simulink model "windyBBBB_sim"  (R2022a)
settings: Solver=FixedStepDiscrete  StartTime=0.0  StopTime=40  FixedStep=0.01  RelTol=1e-3  EnableMultiTasking=on
undefined symbols (not defined in the file or in its folder): sigbuilder_block
libraries: simulink x12, simulink_extras x8
settings Model: PacingRate=0.100000  Creator=Lab  LastModifiedBy=Lab
settings SolverCC: AlgebraicLoopSolver=TrustRegion  AutoInsertRateTranBlk=on
settings DataIOCC: LimitDataPoints=on
settings OptimizationCC: LifeSpan=inf
settings DebuggingCC: UnconnectedInputMsg=warning  UnconnectedOutputMsg=warning  UnconnectedLineMsg=warning  AllowSymbolicDim=off  SFUnexpectedBacktrackingDiag=warning  SFNoUnconditionalDefaultTransitionDiag=warning  SFExecutionAtInitializationDiag=none  ArithmeticOperatorsInVariantConditions=warning
settings SFSimCC: SimUseLocalCustomCode=off  CustomCodeUndefinedFunction=UseInterfaceOnly
settings RTWCC: RTWUseLocalCustomCode=off  DLArmComputeVersion=19.05
settings CodeAppCC: StateflowObjectComments=on
settings GRTTargetCC: TargetLangStandard=C89/C90 (ANSI)
settings ConfigComp: CovMetricSettings=dw  CovSaveCumulativeToWorkspaceVar=on  CovSaveSingleToWorkspaceVar=on  CovExternalEMLEnable=off  CovSFcnEnable=off

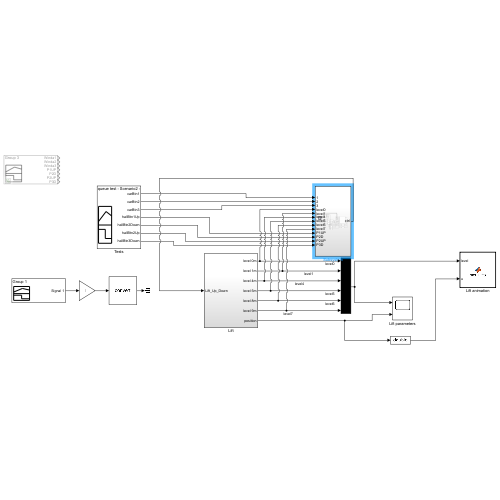
[thumbnail: Simulink's stored preview of the top-level diagram]
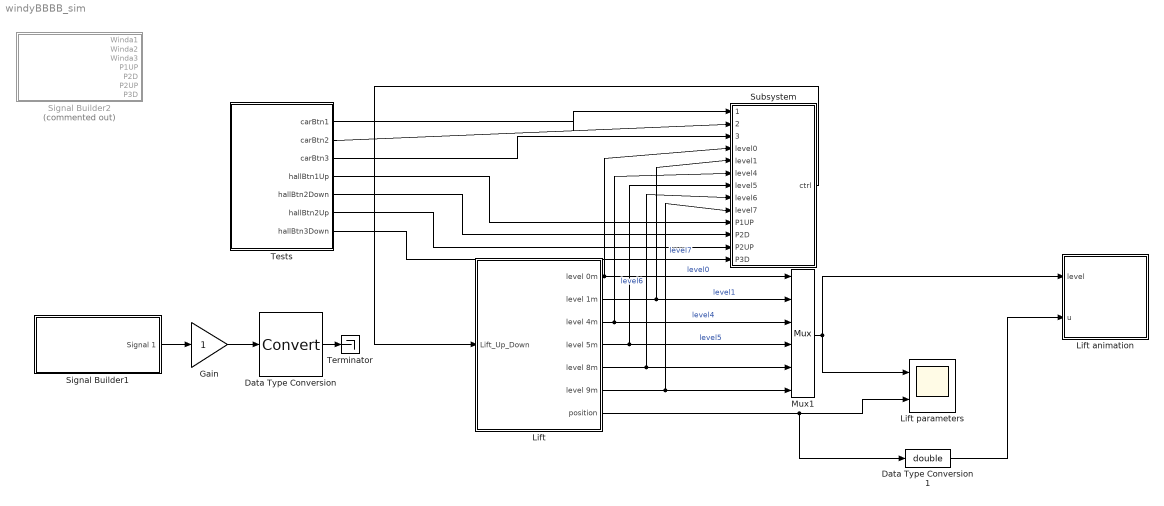
== system windyBBBB_sim ==
  Data Type Conversion : DataTypeConversion  SaturateOnIntegerOverflow=off  RndMeth=Floor
  Data Type Conversion1 : DataTypeConversion  OutDataTypeStr=double  SaturateOnIntegerOverflow=off  RndMeth=Floor
  Gain : Gain
  Lift : Subsystem
  Lift animation : MATLAB Function  TreatAsAtomicUnit=on  SystemSampleTime=0.05
  Lift parameters : Scope  NumInputPorts=2
  Mux1 : Mux  Inputs=6
  Signal Builder1 : Subsystem  Tag=STV Subsys  LoadFcn=sigbuilder_block('load');  StartFcn=sigbuilder_block('start');  StopFcn=sigbuilder_block('stop');  ClipboardFcn=sigbuilder_block('clipboard');  mask(Sigbuilder block){tuvar=[0:10]}
      mask help: Simulink:masks:SigbuilderBlock_MD
      mask init:
      | if ~strcmp(get_param(bdroot(gcbh),'SimulationStatus'),'stopped') tuvar = sigbuilder_block('maskInit'); end
      settings: CopyFcn=sigbuilder_block('copy');  DeleteFcn=sigbuilder_block('delete');  ModelCloseFcn=sigbuilder_block('modelClose');  PreSaveFcn=sigbuilder_block('preSave');  PauseFcn=sigbuilder_block('pause');  ContinueFcn=sigbuilder_block('continue');  NameChangeFcn=sigbuilder_block('namechange');  OpenFcn=sigbuilder_block('open',[327.75 241.5 550.5 394.5 ]);  CloseFcn=sigbuilder_block('close');
      mask Display: plot(0, 0, 100, 100,[2, 2, 32, 32, 2], [68, 8, 8, 68, 68],[32, 2], [38, 38], [32, 19, 2],[53, 60, 44], [32, 17, 17, 2],[16, 16, 31, 31]);txt = getActiveGroup(gcbh);text(2, 100, txt,'verticalAlignment', 'top');
  Signal Builder2 : Subsystem  Tag=STV Subsys  Commented=on  LoadFcn=sigbuilder_block('load');  StartFcn=sigbuilder_block('start');  StopFcn=sigbuilder_block('stop');  ClipboardFcn=sigbuilder_block('clipboard');  mask(Sigbuilder block){tuvar=[0:10]}
      mask help: Simulink:masks:SigbuilderBlock_MD
      mask init:
      | if ~strcmp(get_param(bdroot(gcbh),'SimulationStatus'),'stopped') tuvar = sigbuilder_block('maskInit'); end
      settings: CopyFcn=sigbuilder_block('copy');  DeleteFcn=sigbuilder_block('delete');  ModelCloseFcn=sigbuilder_block('modelClose');  PreSaveFcn=sigbuilder_block('preSave');  PauseFcn=sigbuilder_block('pause');  ContinueFcn=sigbuilder_block('continue');  NameChangeFcn=sigbuilder_block('namechange');  OpenFcn=sigbuilder_block('open',[-1440 -60 1440 723.6 ]);  CloseFcn=sigbuilder_block('close');
      mask Display: plot(0, 0, 100, 100,[2, 2, 32, 32, 2], [68, 8, 8, 68, 68],[32, 2], [38, 38], [32, 19, 2],[53, 60, 44], [32, 17, 17, 2],[16, 16, 31, 31]);txt = getActiveGroup(gcbh);text(2, 100, txt,'verticalAlignment', 'top');
  Subsystem : Subsystem
  Terminator : Terminator
  Tests : Subsystem  Tag=STV Subsys  LoadFcn=sigbuilder_block('load',[-1440 -60 1440 723.6 ]);  StartFcn=sigbuilder_block('start');  StopFcn=sigbuilder_block('stop');  ClipboardFcn=sigbuilder_block('clipboard');  mask(Sigbuilder block){tuvar=[0:10]}
      mask help: Simulink:masks:SigbuilderBlock_MD
      mask init:
      | if ~strcmp(get_param(bdroot(gcbh),'SimulationStatus'),'stopped') tuvar = sigbuilder_block('maskInit'); end
      settings: CopyFcn=sigbuilder_block('copy');  DeleteFcn=sigbuilder_block('delete');  ModelCloseFcn=sigbuilder_block('modelClose');  PreSaveFcn=sigbuilder_block('preSave');  PauseFcn=sigbuilder_block('pause');  ContinueFcn=sigbuilder_block('continue');  NameChangeFcn=sigbuilder_block('namechange');  OpenFcn=sigbuilder_block('open',[9.6 82.8 575.4 499.8 ]);  CloseFcn=sigbuilder_block('close');
      mask Display: plot(0, 0, 100, 100,[2, 2, 32, 32, 2], [68, 8, 8, 68, 68],[32, 2], [38, 38], [32, 19, 2],[53, 60, 44], [32, 17, 17, 2],[16, 16, 31, 31]);txt = getActiveGroup(gcbh);text(2, 100, txt,'verticalAlignment', 'top');
  wires:
  Lift/6(level 9m) -> Subsystem/9(level7), Mux1/6  "level7"
  Lift/2(level 1m) -> Subsystem/5(level1), Mux1/2  "level1"
  Data Type Conversion1/1 -> Lift animation/2(u)
  Lift/7(position) -> Data Type Conversion1/1, Lift parameters/2
  Mux1/1 -> Lift parameters/1, Lift animation/1(level)
  Lift/4(level 5m) -> Subsystem/7(level5), Mux1/4  "level5"
  Gain/1 -> Data Type Conversion/1
  Lift/5(level 8m) -> Subsystem/8(level6), Mux1/5  "level6"
  Signal Builder1/1(Signal 1) -> Gain/1
  Lift/1(level 0m) -> Subsystem/4(level0), Mux1/1  "level0"
  Lift/3(level 4m) -> Subsystem/6(level4), Mux1/3  "level4"
  Data Type Conversion/1 -> Terminator/1
  Tests/1(carBtn1) -> Subsystem/1(1)
  Tests/2(carBtn2) -> Subsystem/2(2)
  Tests/3(carBtn3) -> Subsystem/3(3)
  Subsystem/1(ctrl) -> Lift/1(Lift_Up_Down)
  Tests/4(hallBtn1Up) -> Subsystem/10(P1UP)
  Tests/5(hallBtn2Down) -> Subsystem/11(P2D)
  Tests/6(hallBtn2Up) -> Subsystem/12(P2UP)
  Tests/7(hallBtn3Down) -> Subsystem/13(P3D)

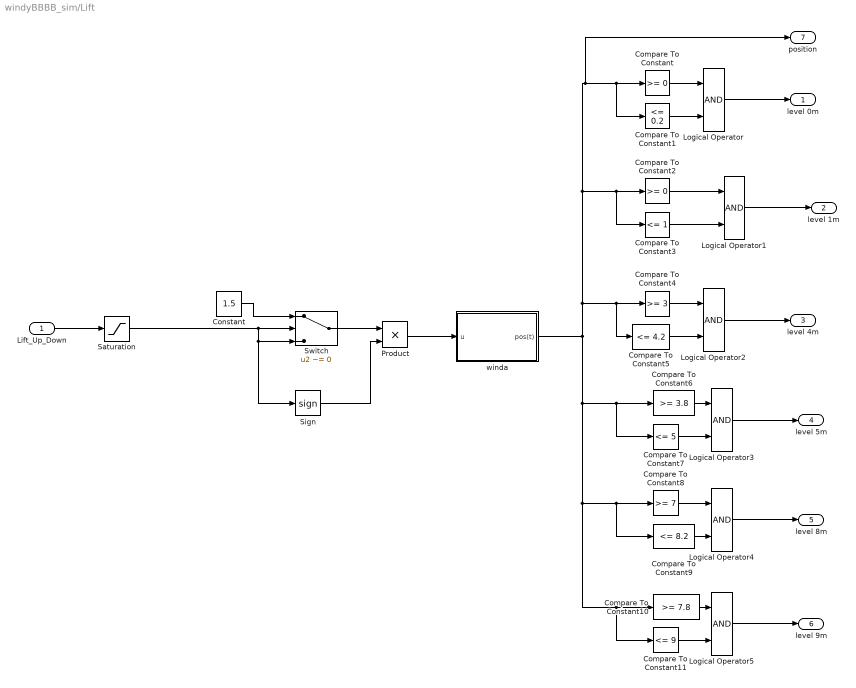
== system windyBBBB_sim/Lift ==
  Lift_Up_Down : Inport
  Compare To Constant : simulink/Logic and Bit Operations/Compare To Constant  relop=>=  const=0  OutDataTypeStr=boolean
  Compare To Constant1 : simulink/Logic and Bit Operations/Compare To Constant  relop=<=  const=0.2  OutDataTypeStr=boolean
  Compare To Constant10 : simulink/Logic and Bit Operations/Compare To Constant  relop=>=  const=7.8  OutDataTypeStr=boolean
  Compare To Constant11 : simulink/Logic and Bit Operations/Compare To Constant  relop=<=  const=9  OutDataTypeStr=boolean
  Compare To Constant2 : simulink/Logic and Bit Operations/Compare To Constant  relop=>=  const=0  OutDataTypeStr=boolean
  Compare To Constant3 : simulink/Logic and Bit Operations/Compare To Constant  relop=<=  const=1  OutDataTypeStr=boolean
  Compare To Constant4 : simulink/Logic and Bit Operations/Compare To Constant  relop=>=  const=3  OutDataTypeStr=boolean
  Compare To Constant5 : simulink/Logic and Bit Operations/Compare To Constant  relop=<=  const=4.2  OutDataTypeStr=boolean
  Compare To Constant6 : simulink/Logic and Bit Operations/Compare To Constant  relop=>=  const=3.8  OutDataTypeStr=boolean
  Compare To Constant7 : simulink/Logic and Bit Operations/Compare To Constant  relop=<=  const=5  OutDataTypeStr=boolean
  Compare To Constant8 : simulink/Logic and Bit Operations/Compare To Constant  relop=>=  const=7  OutDataTypeStr=boolean
  Compare To Constant9 : simulink/Logic and Bit Operations/Compare To Constant  relop=<=  const=8.2  OutDataTypeStr=boolean
  Constant : Constant  Value=1.5
  Logical Operator{,1..5} (6 alike) : Logic  AllPortsSameDT=off  OutDataTypeStr=boolean
  Product : Product  OutDataTypeStr=Inherit: Inherit via back propagation  RndMeth=Zero
  Saturation : Saturate  UpperLimit=1  LowerLimit=-1
  Sign : Signum
  Switch : Switch  Criteria=u2 ~= 0  OutDataTypeStr=Inherit: Inherit via back propagation  SaturateOnIntegerOverflow=off  InputSameDT=off
  winda : Subsystem
  level 0m : Outport
  level 1m : Outport  Port=2
  level 4m : Outport  Port=3
  level 5m : Outport  Port=4
  level 8m : Outport  Port=5
  level 9m : Outport  Port=6
  position : Outport  Port=7
  wires:
  Constant/1 -> Switch/1
  Lift_Up_Down/1 -> Saturation/1
  Switch/1 -> Product/1
  Product/1 -> winda/1(u)
  Sign/1 -> Product/2
  Logical Operator/1 -> level 0m/1
  Compare To Constant/1 -> Logical Operator/1
  Compare To Constant1/1 -> Logical Operator/2
  Logical Operator1/1 -> level 1m/1
  Compare To Constant2/1 -> Logical Operator1/1
  Compare To Constant3/1 -> Logical Operator1/2
  Logical Operator2/1 -> level 4m/1
  Compare To Constant4/1 -> Logical Operator2/1
  Compare To Constant5/1 -> Logical Operator2/2
  Logical Operator3/1 -> level 5m/1
  Compare To Constant6/1 -> Logical Operator3/1
  Compare To Constant7/1 -> Logical Operator3/2
  Logical Operator4/1 -> level 8m/1
  Compare To Constant8/1 -> Logical Operator4/1
  Compare To Constant9/1 -> Logical Operator4/2
  Logical Operator5/1 -> level 9m/1
  winda/1(pos(t)) -> position/1, Compare To Constant1/1, Compare To Constant/1, Compare To Constant2/1, Compare To Constant3/1, Compare To Constant5/1, Compare To Constant4/1, Compare To Constant10/1, Compare To Constant11/1, Compare To Constant9/1, Compare To Constant8/1, Compare To Constant6/1, Compare To Constant7/1
  Compare To Constant10/1 -> Logical Operator5/1
  Compare To Constant11/1 -> Logical Operator5/2
  Saturation/1 -> Sign/1, Switch/3, Switch/2

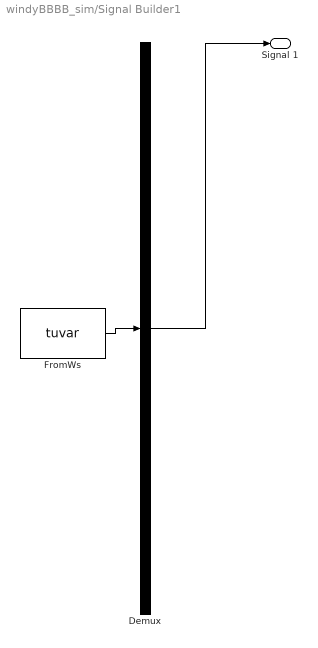
== system windyBBBB_sim/Signal Builder1 ==
  Demux : Demux  Tag=STV Demux  Outputs=1
      settings: DisplayOption=none
  FromWs : FromWorkspace  Tag=STV FromWs  VariableName=tuvar
      SigBuilderData=|
      | common.afterFinalStr = 'Extrapolate'
      | common.sampleTime = 0
      | dataSet.timeRange = [0 40]
      | dataSet.name = 'Group 1'
      | sbobj.Groups.Name = 'Group 1'
      | sbobj.Groups.Signals.Name = 'Signal 1'
      | sbobj.Groups.Signals.XData = [0 10 10 20.1 20.1 30 30 40]
      | sbobj.Groups.Signals.YData = [0 0 0.99 0.99 0 0 -1 -1]
      | sbobj.Groups.TimeRange = [0 40]
  Signal 1 : Outport  Tag=STV Outport
  wires:
  Demux/1 -> Signal 1/1
  FromWs/1 -> Demux/1

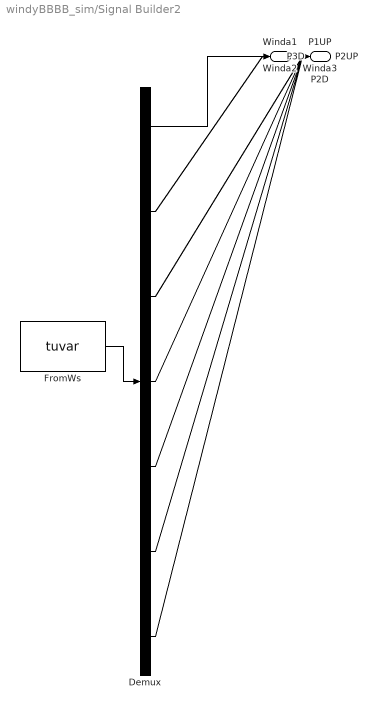
== system windyBBBB_sim/Signal Builder2 ==
  Demux : Demux  Tag=STV Demux  Outputs=7
      settings: DisplayOption=none
  FromWs : FromWorkspace  Tag=STV FromWs  VariableName=tuvar
      SigBuilderData=|
      | common.afterFinalStr = 'Extrapolate'
      | common.sampleTime = 0
      | dataSet(1).timeRange = [0 40]
      | dataSet(1).name = 'Group 1'
      | dataSet(2).timeRange = [0 40]
      | dataSet(2).name = 'Group 2'
      | dataSet(3).timeRange = [0 40]
      | dataSet(3).name = 'Group 3'
      | sbobj.Groups(1).Name = 'Group 1'
      | sbobj.Groups(1).Signals(1).Name = 'Winda1'
      | sbobj.Groups(1).Signals(1).XData = [0 2.4 7.6 10 10 11.25 11.25 40]
      | sbobj.Groups(1).Signals(1).YData = [0 0 0 0 1 1 0 0]
      | sbobj.Groups(1).Signals(2).Name = 'Winda2'
      | sbobj.Groups(1).Signals(2).XData = [0 1.65 1.65 2 2 11.7 11.7 12.8 12.8 30.1 31 40]
      | sbobj.Groups(1).Signals(2).YData = [0 0 1 1 0 0 1 1 0 0 0 0]
      | sbobj.Groups(1).Signals(3).Name = 'Winda3'
      | sbobj.Groups(1).Signals(3).XData = [0 10 10 11.2 11.2 21.9 21.9 23.1 23.1 40]
      | sbobj.Groups(1).Signals(3).YData = [0 0 1 1 0 0 1 1 0 0]
      | sbobj.Groups(1).Signals(4).Name = 'P1UP'
      | sbobj.Groups(1).Signals(4).XData = [0 1.3 2.9 40]
      | sbobj.Groups(1).Signals(4).YData = [0 0 0 0]
      | sbobj.Groups(1).Signals(5).Name = 'P2D'
      | sbobj.Groups(1).Signals(5).XData = [0 35.9 37.4 40]
      | sbobj.Groups(1).Signals(5).YData = [0 0 0 0]
      | sbobj.Groups(1).Signals(6).Name = 'P2UP'
      | sbobj.Groups(1).Signals(6).XData = [0 25.2 26.4 40]
      | sbobj.Groups(1).Signals(6).YData = [0 0 0 0]
      | sbobj.Groups(1).Signals(7).Name = 'P3D'
      | sbobj.Groups(1).Signals(7).XData = [0 35.1 36.3 40]
      | sbobj.Groups(1).Signals(7).YData = [0 0 0 0]
      | sbobj.Groups(1).TimeRange = [0 40]
      | sbobj.Groups(2).Name = 'Group 2'
      | sbobj.Groups(2).Signals(1).Name = 'Winda1'
      | sbobj.Groups(2).Signals(1).XData = [0 2.4 7.6 16.7 16.7 17.3 17.3 40]
      | sbobj.Groups(2).Signals(1).YData = [0 0 0 0 1 1 0 0]
      | sbobj.Groups(2).Signals(2).Name = 'Winda2'
      | sbobj.Groups(2).Signals(2).XData = [0 2.15 2.15 2.4 2.4 17.65 17.65 18.25 18.25 30.1 31 40]
      | sbobj.Groups(2).Signals(2).YData = [0 0 1 1 0 0 1 1 0 0 0 0]
      | sbobj.Groups(2).Signals(3).Name = 'Winda3'
      | sbobj.Groups(2).Signals(3).XData = [0 1.35 1.35 1.6 1.6 21.9 23.1 40]
      | sbobj.Groups(2).Signals(3).YData = [0 0 1 1 0 0 0 0]
      | sbobj.Groups(2).Signals(4).Name = 'P1UP'
      | sbobj.Groups(2).Signals(4).XData = [0 1.3 2.9 40]
      | sbobj.Groups(2).Signals(4).YData = [0 0 0 0]
      | sbobj.Groups(2).Signals(5).Name = 'P2D'
      | sbobj.Groups(2).Signals(5).XData = [0 35.9 37.4 40]
      | sbobj.Groups(2).Signals(5).YData = [0 0 0 0]
      | sbobj.Groups(2).Signals(6).Name = 'P2UP'
      | sbobj.Groups(2).Signals(6).XData = [0 25.2 26.4 40]
      | sbobj.Groups(2).Signals(6).YData = [0 0 0 0]
      | sbobj.Groups(2).Signals(7).Name = 'P3D'
      | sbobj.Groups(2).Signals(7).XData = [0 35.1 36.3 40]
      | sbobj.Groups(2).Signals(7).YData = [0 0 0 0]
      | sbobj.Groups(2).TimeRange = [0 40]
      | sbobj.Groups(3).Name = 'Group 3'
      | sbobj.Groups(3).Signals(1).Name = 'Winda1'
      | sbobj.Groups(3).Signals(1).XData = [0 2.4 7.6 16.7 16.7 17.3 17.3 40]
      | sbobj.Groups(3).Signals(1).YData = [0 0 0 0 1 1 0 0]
      | sbobj.Groups(3).Signals(2).Name = 'Winda2'
      | sbobj.Groups(3).Signals(2).XData = [0 6.4 10.9 17.65 18.25 30.1 31 40]
      | sbobj.Groups(3).Signals(2).YData = [0 0 0 0 0 0 0 0]
      | sbobj.Groups(3).Signals(3).Name = 'Winda3'
      | sbobj.Groups(3).Signals(3).XData = [0 1.35 1.35 1.6 1.6 21.9 23.1 40]
      | sbobj.Groups(3).Signals(3).YData = [0 0 1 1 0 0 0 0]
      | sbobj.Groups(3).Signals(4).Name = 'P1UP'
      | sbobj.Groups(3).Signals(4).XData = [0 1.3 2.9 40]
      | sbobj.Groups(3).Signals(4).YData = [0 0 0 0]
      | sbobj.Groups(3).Signals(5).Name = 'P2D'
      | sbobj.Groups(3).Signals(5).XData = [0 35.9 37.4 40]
      | sbobj.Groups(3).Signals(5).YData = [0 0 0 0]
      | sbobj.Groups(3).Signals(6).Name = 'P2UP'
      | sbobj.Groups(3).Signals(6).XData = [0 25.2 26.4 40]
      | sbobj.Groups(3).Signals(6).YData = [0 0 0 0]
      | sbobj.Groups(3).Signals(7).Name = 'P3D'
      | sbobj.Groups(3).Signals(7).XData = [0 35.1 36.3 40]
      | sbobj.Groups(3).Signals(7).YData = [0 0 0 0]
      | sbobj.Groups(3).TimeRange = [0 40]
  Winda1 : Outport  Tag=STV Outport
  Winda2 : Outport  Tag=STV Outport  Port=2
  Winda3 : Outport  Tag=STV Outport  Port=3
  P1UP : Outport  Tag=STV Outport  Port=4
  P2D : Outport  Tag=STV Outport  Port=5
  P2UP : Outport  Tag=STV Outport  Port=6
  P3D : Outport  Tag=STV Outport  Port=7
  wires:
  FromWs/1 -> Demux/1
  Demux/1 -> Winda1/1
  Demux/2 -> Winda2/1
  Demux/3 -> Winda3/1
  Demux/4 -> P1UP/1
  Demux/5 -> P2D/1
  Demux/6 -> P2UP/1
  Demux/7 -> P3D/1

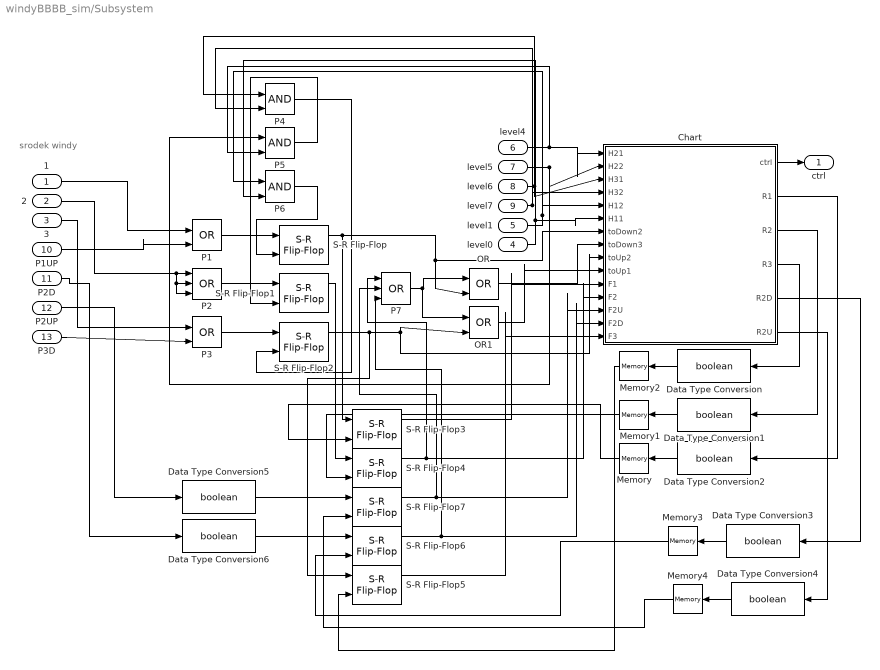
== system windyBBBB_sim/Subsystem ==
  note: srodek windy
  1 : Inport
  2 : Inport  Port=2
  3 : Inport  Port=3
  level0 : Inport  Port=4
  level1 : Inport  Port=5
  level4 : Inport  Port=6
  level5 : Inport  Port=7
  level6 : Inport  Port=8
  level7 : Inport  Port=9
  P1UP : Inport  Port=10
  P2D : Inport  Port=11
  P2UP : Inport  Port=12
  P3D : Inport  Port=13
  Chart : Stateflow chart  TreatAsAtomicUnit=on
      settings: PortSchema="{\"entries\":[{\"content\":{\"sides\":[{\"content\":{\"connectorIds\":[\"In1\",\"In2\",\"In3\",\"In4\",\"In5\",\"In6\",\"In7\",\"In8\",\"In9\",\"In10\",\"In11\",\"In15\",\"In12\",\"In13\",\"In14\"]},\"type\":\"ConnectorPlacement.EquallySpacedRectSide\",\"uuid\":\"c52c96df-b6a3-421e-822c-63f52c3e4f44\"},{\"content\":{\"connectorIds\":[\"Out1\",\"Out2\",\"Out3\",\"Out4\",\"Out5\",\"Out6\"],\"side\":\"RIGHT\"},\"type\":\"ConnectorPlacement.EquallySpacedRectSide\",\"uuid\":\"aa3b0e8d-89ba-4755-a611-2dfadbbaa4ad\"},{\"content\":{\"connectorIds\":[],\"side\":\"TOP\"},\"type\":\"ConnectorPlacement.EquallySpacedRectSide\",\"uuid\":\"c0db1b70-eab9-474d-bd3f-3f1f196ed625\"}]},\"type\":\"ConnectorPlacement.EquallySpacedConnector\",\"uuid\":\"3f6306b3-4465-4ee0-952c-4ab87b7a638d\"}],\"packageUris\":[\"http://schema.mathworks.com/mf0/Connector/R2020b\"],\"version\":\"1.0\"}"
  Data Type Conversion{,1..6} (7 alike) : DataTypeConversion  OutDataTypeStr=boolean  SaturateOnIntegerOverflow=off  RndMeth=Floor
  Memory{,1..4} (5 alike) : Memory
  OR : Logic  Operator=OR  IconShape=distinctive  AllPortsSameDT=off  OutDataTypeStr=boolean
  OR1 : Logic  Operator=OR  IconShape=distinctive  AllPortsSameDT=off  OutDataTypeStr=boolean
  P1 : Logic  Operator=OR  IconShape=distinctive  AllPortsSameDT=off  OutDataTypeStr=boolean
  P2 : Logic  Operator=OR  Inputs=3  IconShape=distinctive  AllPortsSameDT=off  OutDataTypeStr=boolean
  P3 : Logic  Operator=OR  IconShape=distinctive  AllPortsSameDT=off  OutDataTypeStr=boolean
  P4 : Logic  IconShape=distinctive  AllPortsSameDT=off  OutDataTypeStr=boolean
  P5 : Logic  IconShape=distinctive  AllPortsSameDT=off  OutDataTypeStr=boolean
  P6 : Logic  IconShape=distinctive  AllPortsSameDT=off  OutDataTypeStr=boolean
  P7 : Logic  Operator=OR  Inputs=3  IconShape=distinctive  AllPortsSameDT=off  OutDataTypeStr=boolean
  S-R Flip-Flop{,1..7} (8 alike) : simulink_extras/Flip Flops/S-R Flip-Flop  initial_condition=0
  ctrl : Outport
  wires:
  level0/1 -> P6/2, Chart/6(H11)
  S-R Flip-Flop1/1 -> S-R Flip-Flop4/1
  level6/1 -> P4/1, Chart/3(H31)
  OR1/1 -> Chart/10(toUp1)
  OR/1 -> Chart/8(toDown3)
  S-R Flip-Flop/1 -> S-R Flip-Flop3/1, OR/2, Chart/7(toDown2)
  S-R Flip-Flop2/1 -> S-R Flip-Flop5/1, OR1/2, Chart/9(toUp2)
  level4/1 -> P5/2, Chart/1(H21)
  level5/1 -> P5/1, Chart/2(H22)
  level1/1 -> P6/1, Chart/5(H12)
  level7/1 -> P4/2, Chart/4(H32)
  Chart/1(ctrl) -> ctrl/1
  1/1 -> P1/1
  2/1 -> P2/3, P2/2, P2/1
  3/1 -> P3/1
  P1UP/1 -> P1/2
  P2D/1 -> Data Type Conversion6/1
  P2UP/1 -> Data Type Conversion5/1
  P3D/1 -> P3/2
  P1/1 -> S-R Flip-Flop/1
  P2/1 -> S-R Flip-Flop1/1
  P3/1 -> S-R Flip-Flop2/1
  P6/1 -> S-R Flip-Flop/2
  P5/1 -> S-R Flip-Flop1/2
  P4/1 -> S-R Flip-Flop2/2
  Chart/4(R3) -> Data Type Conversion/1
  Data Type Conversion/1 -> Memory2/1
  Chart/3(R2) -> Data Type Conversion1/1
  Chart/2(R1) -> Data Type Conversion2/1
  Data Type Conversion1/1 -> Memory1/1
  Data Type Conversion2/1 -> Memory/1
  Memory/1 -> S-R Flip-Flop3/2
  Memory1/1 -> S-R Flip-Flop4/2
  Memory2/1 -> S-R Flip-Flop5/2
  S-R Flip-Flop3/1 -> Chart/11(F1)
  S-R Flip-Flop4/1 -> P7/1, Chart/15(F2)
  S-R Flip-Flop5/1 -> Chart/14(F3)
  S-R Flip-Flop7/1 -> P7/2, Chart/12(F2U)
  S-R Flip-Flop6/1 -> P7/3, Chart/13(F2D)
  Data Type Conversion3/1 -> Memory3/1
  Data Type Conversion4/1 -> Memory4/1
  Chart/6(R2U) -> Data Type Conversion4/1
  Memory4/1 -> S-R Flip-Flop7/2
  Chart/5(R2D) -> Data Type Conversion3/1
  Memory3/1 -> S-R Flip-Flop6/2
  Data Type Conversion5/1 -> S-R Flip-Flop7/1
  Data Type Conversion6/1 -> S-R Flip-Flop6/1
  P7/1 -> OR1/1, OR/1

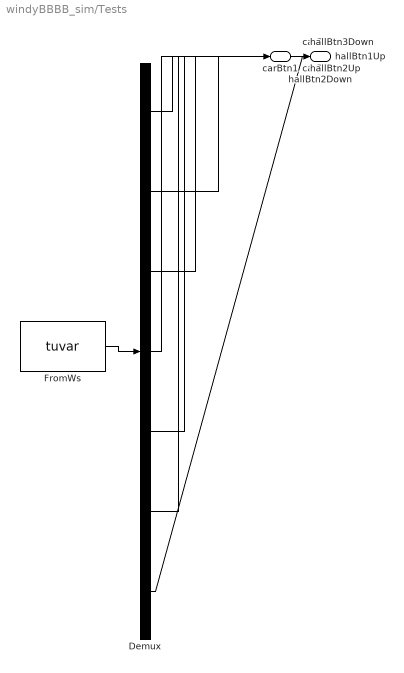
== system windyBBBB_sim/Tests ==
  Demux : Demux  Tag=STV Demux  Outputs=7
      settings: DisplayOption=none
  FromWs : FromWorkspace  Tag=STV FromWs  VariableName=tuvar
      SigBuilderData=|
      | common.afterFinalStr = 'Extrapolate'
      | common.sampleTime = 0
      | dataSet(1).timeRange = [0 40]
      | dataSet(1).name = 'carBtns test'
      | dataSet(2).timeRange = [0 40]
      | dataSet(2).name = 'hallBtns test'
      | dataSet(3).timeRange = [0 40]
      | dataSet(3).name = 'queue test - Scenario1 - insert in the middle'
      | dataSet(4).timeRange = [0 40]
      | dataSet(4).name = 'queue test - Scenario1 - insert at the end'
      | dataSet(5).timeRange = [0 40]
      | dataSet(5).name = 'queue test - Scenario2 - inset at the end'
      | dataSet(6).timeRange = [0 40]
      | dataSet(6).name = 'dziwna_sytuacja'
      | sbobj.Groups(1).Name = 'carBtns test'
      | sbobj.Groups(1).Signals(1).Name = 'carBtn1'
      | sbobj.Groups(1).Signals(1).XData = [0 13 13 14 14 40]
      | sbobj.Groups(1).Signals(1).YData = [0 0 1 1 0 0]
      | sbobj.Groups(1).Signals(2).Name = 'carBtn2'
      | sbobj.Groups(1).Signals(2).XData = [0 3 3 4 4 40]
      | sbobj.Groups(1).Signals(2).YData = [0 0 1 1 0 0]
      | sbobj.Groups(1).Signals(3).Name = 'carBtn3'
      | sbobj.Groups(1).Signals(3).XData = [0 8 8 9 9 40]
      | sbobj.Groups(1).Signals(3).YData = [0 0 1 1 0 0]
      | sbobj.Groups(1).Signals(4).Name = 'hallBtn1Up'
      | sbobj.Groups(1).Signals(4).XData = [0 16 24 40]
      | sbobj.Groups(1).Signals(4).YData = [0 0 0 0]
      | sbobj.Groups(1).Signals(5).Name = 'hallBtn2Down'
      | sbobj.Groups(1).Signals(5).XData = [0 16 24 40]
      | sbobj.Groups(1).Signals(5).YData = [0 0 0 0]
      | sbobj.Groups(1).Signals(6).Name = 'hallBtn2Up'
      | sbobj.Groups(1).Signals(6).XData = [0 16 24 40]
      | sbobj.Groups(1).Signals(6).YData = [0 0 0 0]
      | sbobj.Groups(1).Signals(7).Name = 'hallBtn3Down'
      | sbobj.Groups(1).Signals(7).XData = [0 16 24 40]
      | sbobj.Groups(1).Signals(7).YData = [0 0 0 0]
      | sbobj.Groups(1).TimeRange = [0 40]
      | sbobj.Groups(2).Name = 'hallBtns test'
      | sbobj.Groups(2).Signals(1).Name = 'carBtn1'
      | sbobj.Groups(2).Signals(1).XData = [0 13 14 40]
      | sbobj.Groups(2).Signals(1).YData = [0 0 0 0]
      | sbobj.Groups(2).Signals(2).Name = 'carBtn2'
      | sbobj.Groups(2).Signals(2).XData = [0 3 4 40]
      | sbobj.Groups(2).Signals(2).YData = [0 0 0 0]
      | sbobj.Groups(2).Signals(3).Name = 'carBtn3'
      | sbobj.Groups(2).Signals(3).XData = [0 8 9 40]
      | sbobj.Groups(2).Signals(3).YData = [0 0 0 0]
      | sbobj.Groups(2).Signals(4).Name = 'hallBtn1Up'
      | sbobj.Groups(2).Signals(4).XData = [0 20 20 21 21 40]
      | sbobj.Groups(2).Signals(4).YData = [0 0 1 1 0 0]
      | sbobj.Groups(2).Signals(5).Name = 'hallBtn2Down'
      | sbobj.Groups(2).Signals(5).XData = [0 25 25 26 26 40]
      | sbobj.Groups(2).Signals(5).YData = [0 0 1 1 0 0]
      | sbobj.Groups(2).Signals(6).Name = 'hallBtn2Up'
      | sbobj.Groups(2).Signals(6).XData = [0 5 5 6 6 40]
      | sbobj.Groups(2).Signals(6).YData = [0 0 1 1 0 0]
      | sbobj.Groups(2).Signals(7).Name = 'hallBtn3Down'
      | sbobj.Groups(2).Signals(7).XData = [0 10 10 11 11 40]
      | sbobj.Groups(2).Signals(7).YData = [0 0 1 1 0 0]
      | sbobj.Groups(2).TimeRange = [0 40]
      | sbobj.Groups(3).Name = 'queue test - Scenario1 - insert in the middle'
      | sbobj.Groups(3).Signals(1).Name = 'carBtn1'
      | sbobj.Groups(3).Signals(1).XData = [0 13 14 40]
      | sbobj.Groups(3).Signals(1).YData = [0 0 0 0]
      | sbobj.Groups(3).Signals(2).Name = 'carBtn2'
      | sbobj.Groups(3).Signals(2).XData = [0 7 7 8 8 40]
      | sbobj.Groups(3).Signals(2).YData = [0 0 1 1 0 0]
      | sbobj.Groups(3).Signals(3).Name = 'carBtn3'
      | sbobj.Groups(3).Signals(3).XData = [0 8 9 40]
      | sbobj.Groups(3).Signals(3).YData = [0 0 0 0]
      | sbobj.Groups(3).Signals(4).Name = 'hallBtn1Up'
      | sbobj.Groups(3).Signals(4).XData = [0 20 21 40]
      | sbobj.Groups(3).Signals(4).YData = [0 0 0 0]
      | sbobj.Groups(3).Signals(5).Name = 'hallBtn2Down'
      | sbobj.Groups(3).Signals(5).XData = [0 25 26 40]
      | sbobj.Groups(3).Signals(5).YData = [0 0 0 0]
      | sbobj.Groups(3).Signals(6).Name = 'hallBtn2Up'
      | sbobj.Groups(3).Signals(6).XData = [0 5 6 40]
      | sbobj.Groups(3).Signals(6).YData = [0 0 0 0]
      | sbobj.Groups(3).Signals(7).Name = 'hallBtn3Down'
      | sbobj.Groups(3).Signals(7).XData = [0 5 5 6 6 40]
      | sbobj.Groups(3).Signals(7).YData = [0 0 1 1 0 0]
      | sbobj.Groups(3).TimeRange = [0 40]
      | sbobj.Groups(4).Name = 'queue test - Scenario1 - insert at the end'
      | sbobj.Groups(4).Signals(1).Name = 'carBtn1'
      | sbobj.Groups(4).Signals(1).XData = [0 13 14 40]
      | sbobj.Groups(4).Signals(1).YData = [0 0 0 0]
      | sbobj.Groups(4).Signals(2).Name = 'carBtn2'
      | sbobj.Groups(4).Signals(2).XData = [0 11 11 12 12 40]
      | sbobj.Groups(4).Signals(2).YData = [0 0 1 1 0 0]
      | sbobj.Groups(4).Signals(3).Name = 'carBtn3'
      | sbobj.Groups(4).Signals(3).XData = [0 8 9 40]
      | sbobj.Groups(4).Signals(3).YData = [0 0 0 0]
      | sbobj.Groups(4).Signals(4).Name = 'hallBtn1Up'
      | sbobj.Groups(4).Signals(4).XData = [0 20 21 40]
      | sbobj.Groups(4).Signals(4).YData = [0 0 0 0]
      | sbobj.Groups(4).Signals(5).Name = 'hallBtn2Down'
      | sbobj.Groups(4).Signals(5).XData = [0 25 26 40]
      | sbobj.Groups(4).Signals(5).YData = [0 0 0 0]
      | sbobj.Groups(4).Signals(6).Name = 'hallBtn2Up'
      | sbobj.Groups(4).Signals(6).XData = [0 5 6 40]
      | sbobj.Groups(4).Signals(6).YData = [0 0 0 0]
      | sbobj.Groups(4).Signals(7).Name = 'hallBtn3Down'
      | sbobj.Groups(4).Signals(7).XData = [0 5 5 6 6 40]
      | sbobj.Groups(4).Signals(7).YData = [0 0 1 1 0 0]
      | sbobj.Groups(4).TimeRange = [0 40]
      | sbobj.Groups(5).Name = 'queue test - Scenario2 - inset at the end'
      | sbobj.Groups(5).Signals(1).Name = 'carBtn1'
      | sbobj.Groups(5).Signals(1).XData = [0 13 14 40]
      | sbobj.Groups(5).Signals(1).YData = [0 0 0 0]
      | sbobj.Groups(5).Signals(2).Name = 'carBtn2'
      | sbobj.Groups(5).Signals(2).XData = [0 6 7 40]
      | sbobj.Groups(5).Signals(2).YData = [0 0 0 0]
      | sbobj.Groups(5).Signals(3).Name = 'carBtn3'
      | sbobj.Groups(5).Signals(3).XData = [0 5 5 6 6 40]
      | sbobj.Groups(5).Signals(3).YData = [0 0 1 1 0 0]
      | sbobj.Groups(5).Signals(4).Name = 'hallBtn1Up'
      | sbobj.Groups(5).Signals(4).XData = [0 20 21 40]
      | sbobj.Groups(5).Signals(4).YData = [0 0 0 0]
      | sbobj.Groups(5).Signals(5).Name = 'hallBtn2Down'
      | sbobj.Groups(5).Signals(5).XData = [0 6.5 6.5 7.5 7.5 40]
      | sbobj.Groups(5).Signals(5).YData = [0 0 1 1 0 0]
      | sbobj.Groups(5).Signals(6).Name = 'hallBtn2Up'
      | sbobj.Groups(5).Signals(6).XData = [0 5 6 40]
      | sbobj.Groups(5).Signals(6).YData = [0 0 0 0]
      | sbobj.Groups(5).Signals(7).Name = 'hallBtn3Down'
      | sbobj.Groups(5).Signals(7).XData = [0 5 6 40]
      | sbobj.Groups(5).Signals(7).YData = [0 0 0 0]
      | sbobj.Groups(5).TimeRange = [0 40]
      | sbobj.Groups(6).Name = 'dziwna_sytuacja'
      | sbobj.Groups(6).Signals(1).Name = 'carBtn1'
      | sbobj.Groups(6).Signals(1).XData = [0 5 6 40]
      | sbobj.Groups(6).Signals(1).YData = [0 0 0 0]
      | sbobj.Groups(6).Signals(2).Name = 'carBtn2'
      | sbobj.Groups(6).Signals(2).XData = [0 6 7 40]
      | sbobj.Groups(6).Signals(2).YData = [0 0 0 0]
      | sbobj.Groups(6).Signals(3).Name = 'carBtn3'
      | sbobj.Groups(6).Signals(3).XData = [0 4 4 5 5 40]
      | sbobj.Groups(6).Signals(3).YData = [0 0 1 1 0 0]
      | sbobj.Groups(6).Signals(4).Name = 'hallBtn1Up'
      | sbobj.Groups(6).Signals(4).XData = [0 20 21 40]
      | sbobj.Groups(6).Signals(4).YData = [0 0 0 0]
      | sbobj.Groups(6).Signals(5).Name = 'hallBtn2Down'
      | sbobj.Groups(6).Signals(5).XData = [0 5.5 5.5 6.5 6.5 40]
      | sbobj.Groups(6).Signals(5).YData = [0 0 1 1 0 0]
      | sbobj.Groups(6).Signals(6).Name = 'hallBtn2Up'
      | sbobj.Groups(6).Signals(6).XData = [0 5.5 5.5 6.5 6.5 40]
      | sbobj.Groups(6).Signals(6).YData = [0 0 1 1 0 0]
      | sbobj.Groups(6).Signals(7).Name = 'hallBtn3Down'
      | sbobj.Groups(6).Signals(7).XData = [0 5 6 40]
      | sbobj.Groups(6).Signals(7).YData = [0 0 0 0]
      | sbobj.Groups(6).TimeRange = [0 40]
  carBtn1 : Outport  Tag=STV Outport
  carBtn2 : Outport  Tag=STV Outport  Port=2
  carBtn3 : Outport  Tag=STV Outport  Port=3
  hallBtn1Up : Outport  Tag=STV Outport  Port=4
  hallBtn2Down : Outport  Tag=STV Outport  Port=5
  hallBtn2Up : Outport  Tag=STV Outport  Port=6
  hallBtn3Down : Outport  Tag=STV Outport  Port=7
  wires:
  Demux/1 -> carBtn1/1
  FromWs/1 -> Demux/1
  Demux/2 -> carBtn2/1
  Demux/3 -> carBtn3/1
  Demux/4 -> hallBtn1Up/1
  Demux/5 -> hallBtn2Down/1
  Demux/6 -> hallBtn2Up/1
  Demux/7 -> hallBtn3Down/1

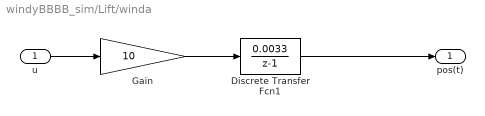
== system windyBBBB_sim/Lift/winda ==
  u : Inport
  Discrete Transfer Fcn1 : DiscreteTransferFcn  Numerator=[0.0033]  Denominator=[1 -1]  SampleTime=0.05  StateDataTypeStr=fixdt(1,26,12)  NumCoefDataTypeStr=fixdt(1,26,12)  DenCoefDataTypeStr=fixdt(1,26,12)  NumProductDataTypeStr=fixdt(1,26,12)  DenProductDataTypeStr=fixdt(1,26,12)  NumAccumDataTypeStr=fixdt(1,26,12)  DenAccumDataTypeStr=fixdt(1,26,12)  OutDataTypeStr=fixdt(1,26,12)
  Gain : Gain  Gain=10  ParamDataTypeStr=fixdt(1,15,2)  OutDataTypeStr=Inherit: Same as input
  pos(t) : Outport
  wires:
  u/1 -> Gain/1
  Gain/1 -> Discrete Transfer Fcn1/1
  Discrete Transfer Fcn1/1 -> pos(t)/1

== matlab function windyBBBB_sim/Lift animation ==
  data: level input; u input
function plot_Lift3( level,u)
%#codegen




persistent fig3;
persistent NOWE1;
persistent L_pos;


if isempty(L_pos),

    if isempty(fig3), 
    fig3 = figure(3);
    else
    close(fig3);
    fig3 = figure(3);
    end
     %NOWE1 = [0 0.1 0.1 0 0; 0.25 .25 0 0 .25]*10;
    NOWE1 = [.1 0 0 .1 .1 .09 .09 .1; 0 0 0.25 0.25 0 0 0.12 .12]*10;
    
    axis([-4 4 -1 15]);
    grid('off');
    %xlabel('X position [m]');
    ylabel('Lift position [m]');
    hold('on');
    line([-0.05 -0.05],[0 12],'LineWidth',2,'Color','k')
    line([1.05 1.05],[0 12],'LineWidth',2,'Color','k')
    line([-4 4],[-0.05 -0.05],'LineWidth',2,'Color','k')
    
    line([-1 -0.05],[4 4],'LineWidth',2,'Color','k')
    line([1.05 2],[4 4],'LineWidth',2,'Color','k')
    
    line([-1 -0.05],[8 8],'LineWidth',2,'Color','k')
    line([1.05 2],[8 8],'LineWidth',2,'Color','k')
    
    line([-1 -0.05],[12 12],'LineWidth',2,'Color','k')
    line([1.05 2],[12 12],'LineWidth',2,'Color','k')
    
 % czarna lampka na wysokosci 0
 line([1.05 1.2],[0.2 0.2],'LineWidth',4,'Color','k')

 % czarna lampka na wysokosci 1
 line([1.05 1.2],[1 1],'LineWidth',4,'Color','k')
    
 % czarna lampka na wysokosci 4
 line([1.05 1.2],[4 4],'LineWidth',4,'Color','k')

 % czarna lampka na wysokosci 5
 line([1.05 1.2],[5 5],'LineWidth',4,'Color','k')
    
  % czarna lampka na wysokosci 8
 line([1.05 1.2],[8 8],'LineWidth',4,'Color','k')
 % czarna lampka na wysokosci 9
 line([1.05 1.2],[9 9],'LineWidth',4,'Color','k')
   
%plot(NOWE1(1,:),NOWE1(2,:)+prev1,'w');
L_pos=plot(NOWE1(1,:),NOWE1(2,:)+u,'b');
    
    
    
else
    if(ishghandle(L_pos)),
       
        set(L_pos,'yData',NOWE1(2,:)+u);
        drawnow limitrate


if level(1)==1    
 % czarna lampka na wysokosci 0
 line([1.05 1.2],[0.2 0.2],'LineWidth',4,'Color','r');
else
 line([1.05 1.2],[0.2 0.2],'LineWidth',4,'Color','k');
end

if level(2)==1    
 % czarna lampka na wysokosci 1
 line([1.05 1.2],[1 1],'LineWidth',4,'Color','r');
else
 line([1.05 1.2],[1 1],'LineWidth',4,'Color','k');
end

if level(3)==1    
 % czarna lampka na wysokosci 4
 line([1.05 1.2],[4 4],'LineWidth',4,'Color','r');
else
 line([1.05 1.2],[4 4],'LineWidth',4,'Color','k');
end

if level(4)==1    
 % czarna lampka na wysokosci 5
 line([1.05 1.2],[5 5],'LineWidth',4,'Color','r');
else
 line([1.05 1.2],[5 5],'LineWidth',4,'Color','k');
end

if level(5)==1    
 % czarna lampka na wysokosci 8
 line([1.05 1.2],[8 8],'LineWidth',4,'Color','r');
else
 line([1.05 1.2],[8 8],'LineWidth',4,'Color','k');
end

if level(6)==1    
 % czarna lampka na wysokosci 9
 line([1.05 1.2],[9 9],'LineWidth',4,'Color','r');
else
 line([1.05 1.2],[9 9],'LineWidth',4,'Color','k');
end



     
        
        
        
    end,
end

== stateflow chart windyBBBB_sim/Subsystem/Chart ==
  state Floor2
    state Go
    state StopD
      ctrl=0;
      %wait
    state resetD
      R2=1;
      R2D=1;
    state StopU
      ctrl=0;
      %wait
    state resetU
      R2=1;
      R2U=1;
    state Stop2
      ctrl=0;
      %wait
    state reset
      R2=1;
    (default) -> Floor2.Go
    Floor2.Go -> StopD [order 1] : [((~F3||F1)&&F2D)]
    StopD -> resetD : after(1, sec)
    Floor2.Go -> Stop2 [order 3] : [F2]
    Floor2.Go -> StopU [order 2] : [((~F1||F3)&&F2U)]
    StopU -> resetU : after(1, sec)
    Stop2 -> Floor2.reset : after(1, sec)
  state Floor3
    state Go
    state Stop
      ctrl=0;
    state reset
      R3=1;
    (default) -> Floor3.Go
    Floor3.Go -> Floor3.Stop : [F3]
    Floor3.Stop -> Floor3.reset : after(1, sec)
  state Floor1
    state Go
    state Stop
      ctrl=0;
    state reset
      R1=1;
    (default) -> Floor1.Go
    Floor1.Go -> Floor1.Stop : [F1]
    Floor1.Stop -> Floor1.reset : after(1, sec)
  state up12
    ctrl=1;
  state up23
    ctrl=1;
  state down21
    ctrl=-1;
  state down32
    ctrl=-1;
  (default) -> Floor1
  Floor1 -> up12 : [toUp1&&~F1]{R1=0}
  up12 -> Floor2 : [H21&&H22]
  Floor2 -> up23 [order 1] : [toUp2&&~F2&&~F2U]{R2=0, R2U=0}
  up23 -> Floor3 : [H31&&H32]
  Floor3 -> down32 : [toDown3&&~F3]{R3=0}
  down21 -> Floor1 : [H11&&H12]
  Floor2 -> down21 [order 2] : [toDown2&&~F2&&~F2D]{R2=0, R2D=0}
  down32 -> Floor2 : [H21&&H22]
  data: H21 input; H22 input; H31 input; H32 input; H12 input; H11 input; toDown2 input; toDown3 input; toUp2 input; toUp1 input; ctrl output; F1 input; F2U input; R1 output; R2 output; R3 output; F2D input; F3 input; F2 input; R2D output; R2U output
